simulink model "Apollo_LM_observer_R2018a"  (R2018a)
settings: Solver=VariableStepAuto  StartTime=0.0  StopTime=60  RelTol=1e-3
model workspace (MATLAB code in the model file):
  | g_M = 1.62; %m/s gravity at moon surface
  | J = 1e5; %kg*m*m
values from neighbouring files (symbols this model uses):
  C = [0,0,1]    [Apollo_LM_design.m]    (also in Apollo_LM_design_observer.m; Apollo_LM_share.m; L11.m = [0,0,2]; cart-oscillator-input-design.m = [1, 0])
  Gamma = h*k1*[1;h/2; k2*h^2/6]    [Apollo_LM_design.m]    (also in Apollo_LM_design_observer.m; Apollo_LM_share.m)
  h = 0.25    [Apollo_LM_design.m]    (also in Apollo_LM_design_observer.m; Apollo_LM_share.m; L11.m = 0.1; cart-oscillator-input-design.m = 0.5)
  K = K_a    [Apollo_LM_design_observer.m]
  L = L_a    [Apollo_LM_design.m]    (also in Apollo_LM_design_observer.m; Apollo_LM_share.m; gantry_crane_equations_of_motion.m = Tt+Tc - V)
  l0 = 1/(C*inv((eye(3)-Phic))*Gamma)    [Apollo_LM_design.m]    (also in Apollo_LM_design_observer.m; Apollo_LM_share.m)
  Phi = [1, 0 , 0 ... (first row only)    [Apollo_LM_design.m]    (also in Apollo_LM_design_observer.m; Apollo_LM_share.m)
settings Model: Creator=kjartan  LastModifiedBy=kjartan
settings SFSimCC: SimUseLocalCustomCode=on
settings RTWCC: RTWUseLocalCustomCode=on

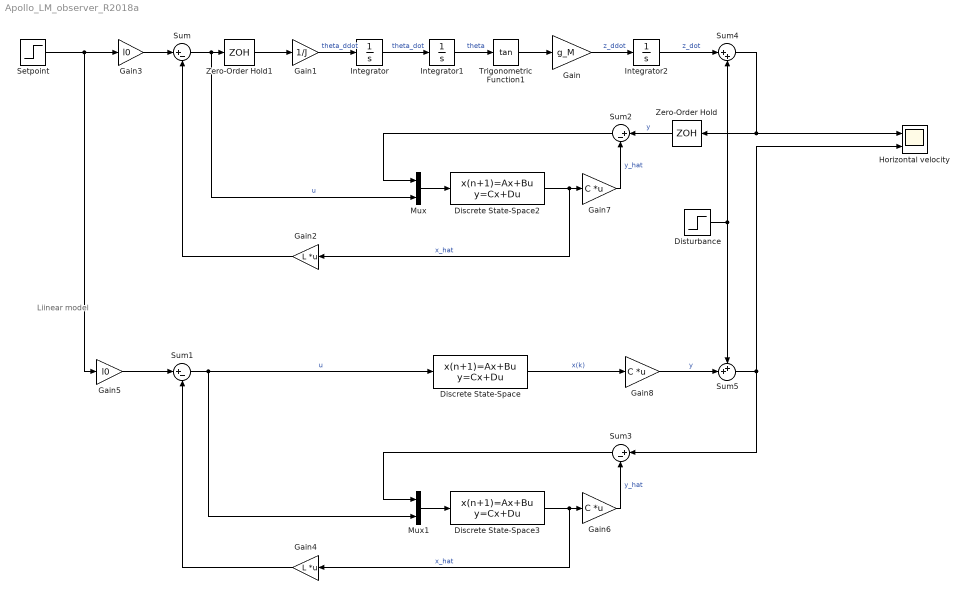
== system Apollo_LM_observer_R2018a ==
  note: Liinear model
  Discrete State-Space : DiscreteStateSpace  A=Phi  B=Gamma  C=eye(3)  D=zeros(3,1)  SampleTime=h
  Discrete State-Space2 : DiscreteStateSpace  A=Phi  B=[K, Gamma]  C=eye(3)  D=zeros(3,2)  SampleTime=h
  Discrete State-Space3 : DiscreteStateSpace  A=Phi  B=[K, Gamma]  C=eye(3)  D=zeros(3,2)  SampleTime=h
  Disturbance : Step  Time=30  SampleTime=0
  Gain : Gain  Gain=g_M
  Gain1 : Gain  Gain=1/J
  Gain2 : Gain  Gain=L  Multiplication=Matrix(K*u)
  Gain3 : Gain  Gain=l0
  Gain4 : Gain  Gain=L  Multiplication=Matrix(K*u)
  Gain5 : Gain  Gain=l0
  Gain6 : Gain  Gain=C  Multiplication=Matrix(K*u)
  Gain7 : Gain  Gain=C  Multiplication=Matrix(K*u)
  Gain8 : Gain  Gain=C  Multiplication=Matrix(K*u)
  Horizontal velocity : Scope  NumInputPorts=2
  Integrator : Integrator
  Integrator1 : Integrator
  Integrator2 : Integrator
  Mux : Mux  Inputs=2
  Mux1 : Mux  Inputs=2
  Setpoint : Step  SampleTime=0
  Sum{,1..3} (4 alike) : Sum  Inputs=|+-
  Sum4 : Sum  Inputs=|++
  Sum5 : Sum  Inputs=++|
  Trigonometric Function1 : Trigonometry  Operator=tan
  Zero-Order Hold : ZeroOrderHold  SampleTime=h
  Zero-Order Hold1 : ZeroOrderHold  SampleTime=h
  wires:
  Integrator1/1 -> Trigonometric Function1/1  "theta"
  Trigonometric Function1/1 -> Gain/1
  Integrator/1 -> Integrator1/1  "theta_dot"
  Gain1/1 -> Integrator/1  "theta_ddot"
  Gain/1 -> Integrator2/1  "z_ddot"
  Sum/1 -> Mux/2, Zero-Order Hold1/1  "u"
  Gain2/1 -> Sum/2
  Gain3/1 -> Sum/1
  Zero-Order Hold1/1 -> Gain1/1
  Discrete State-Space/1 -> Gain8/1  "x(k)"
  Setpoint/1 -> Gain5/1, Gain3/1
  Gain5/1 -> Sum1/1
  Discrete State-Space2/1 -> Gain2/1, Gain7/1  "x_hat"
  Zero-Order Hold/1 -> Sum2/1  "y"
  Gain7/1 -> Sum2/2  "y_hat"
  Sum2/1 -> Mux/1
  Mux/1 -> Discrete State-Space2/1
  Mux1/1 -> Discrete State-Space3/1
  Discrete State-Space3/1 -> Gain4/1, Gain6/1  "x_hat"
  Sum3/1 -> Mux1/1
  Sum1/1 -> Mux1/2, Discrete State-Space/1  "u"
  Gain6/1 -> Sum3/2  "y_hat"
  Gain4/1 -> Sum1/2
  Integrator2/1 -> Sum4/1  "z_dot"
  Disturbance/1 -> Sum5/1, Sum4/2
  Sum4/1 -> Horizontal velocity/1, Zero-Order Hold/1
  Gain8/1 -> Sum5/2  "y"
  Sum5/1 -> Sum3/1, Horizontal velocity/2
